simulink model "SIM001"  (R2019a)
settings: Solver=FixedStepAuto  StartTime=0.0  StopTime=10.0  FixedStep=0.05  RelTol=1e-3
values from neighbouring files (symbols this model uses):
  c = c_st + c_gen    (= 0.1024)    [SIM001.m]    (also in SIM004_DIMENSIONAL_PARAMS.m = 0)
  F0 = rho_w*D*U^2*L*sqrt(2)*CL_rms/2    [SIM001.m]
  fv = St*U/D    [SIM001.m]
  k = 200    [SIM001.m]    (also in SIM002.m = 280; SIM004_DIMENSIONAL_PARAMS.m)
  M = m + m_h    (= 4.82548631591)    [SIM001.m]    (also in SIM002.m = 5.6587609211; SIM004_DIMENSIONAL_PARAMS.m = 5.6587609211)
settings Model: Creator=dinet  LastModifiedBy=dinet

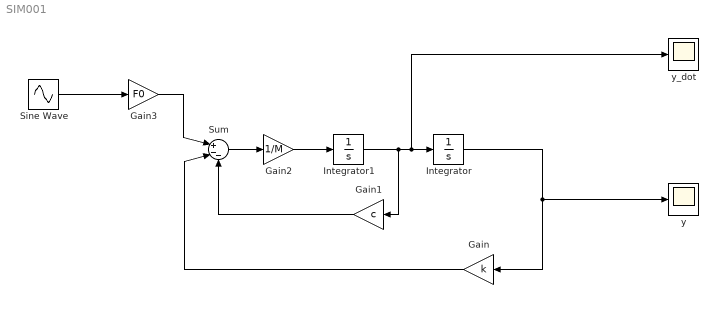
== system SIM001 ==
  Gain : Gain  Gain=k
  Gain1 : Gain  Gain=c
  Gain2 : Gain  Gain=1/M
  Gain3 : Gain  Gain=F0
  Integrator : Integrator
  Integrator1 : Integrator
  Sine Wave : Sin  Frequency=2*pi*fv  SampleTime=0
  Sum : Sum  Inputs=|+--
  y : Scope
  y_dot : Scope
  wires:
  Integrator1/1 -> Gain1/1, y_dot/1, Integrator/1
  Integrator/1 -> y/1, Gain/1
  Gain1/1 -> Sum/3
  Gain/1 -> Sum/2
  Sum/1 -> Gain2/1
  Gain2/1 -> Integrator1/1
  Sine Wave/1 -> Gain3/1
  Gain3/1 -> Sum/1
